simulink model "new_mod"  (Simulink 7.6)
settings: Solver=ode45  StartTime=0.0  StopTime=10.0  RelTol=1e-3
settings Model: Creator=dvaidya  LastModifiedBy=srinrao

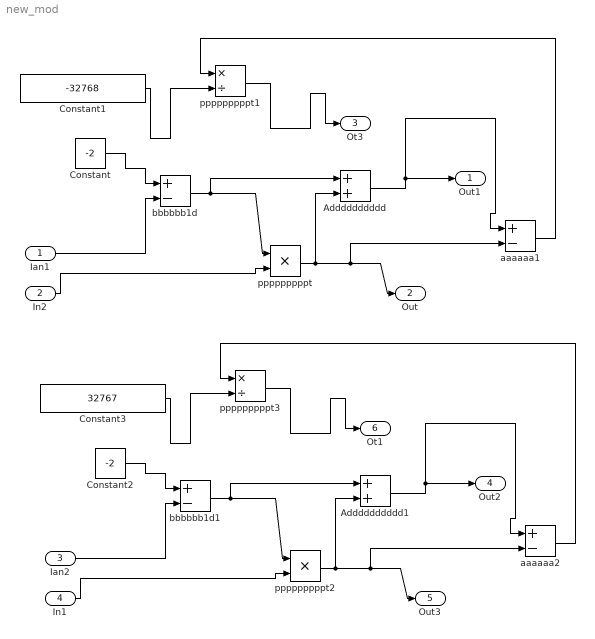
== system new_mod ==
  Ian1 : Inport
  In2 : Inport  Port=2
  Ian2 : Inport  Port=3
  In1 : Inport  Port=4
  Adddddddddd : Sum
  Adddddddddd1 : Sum
  Constant : Constant  Value=-2
  Constant1 : Constant  Value=-32768
  Constant2 : Constant  Value=-2
  Constant3 : Constant  Value=32767
  aaaaaa1 : Sum  Inputs=+-
  aaaaaa2 : Sum  Inputs=+-
  bbbbbb1d : Sum  Inputs=+-
  bbbbbb1d1 : Sum  Inputs=+-
  pppppppppt : Product  RndMeth=Zero
  pppppppppt1 : Product  Inputs=*/  RndMeth=Zero
  pppppppppt2 : Product  RndMeth=Zero
  pppppppppt3 : Product  Inputs=*/  RndMeth=Zero
  Out1 : Outport
  Out : Outport  Port=2
  Ot3 : Outport  Port=3
  Out2 : Outport  Port=4
  Out3 : Outport  Port=5
  Ot1 : Outport  Port=6
  wires:
  Constant/1 -> bbbbbb1d/1
  pppppppppt/1 -> Adddddddddd/2, Out/1, aaaaaa1/2
  Ian1/1 -> bbbbbb1d/2
  In2/1 -> pppppppppt/2
  bbbbbb1d/1 -> Adddddddddd/1, pppppppppt/1
  Adddddddddd/1 -> Out1/1, aaaaaa1/1
  aaaaaa1/1 -> pppppppppt1/1
  Constant1/1 -> pppppppppt1/2
  pppppppppt1/1 -> Ot3/1
  Constant2/1 -> bbbbbb1d1/1
  pppppppppt2/1 -> aaaaaa2/2, Out3/1, Adddddddddd1/2
  Ian2/1 -> bbbbbb1d1/2
  In1/1 -> pppppppppt2/2
  bbbbbb1d1/1 -> pppppppppt2/1, Adddddddddd1/1
  Adddddddddd1/1 -> aaaaaa2/1, Out2/1
  aaaaaa2/1 -> pppppppppt3/1
  Constant3/1 -> pppppppppt3/2
  pppppppppt3/1 -> Ot1/1
